simulink model "propulsionSystem"  (R2019b)
settings: Solver=VariableStepAuto  StartTime=0.0  StopTime=15.0  RelTol=1e-3
undefined symbols (not defined in the file or in its folder): sim
libraries: fl_lib x33, nesl_utility x16, SimscapeFluids_lib x1
settings Model: Creator=Edward  LastModifiedBy=Edward

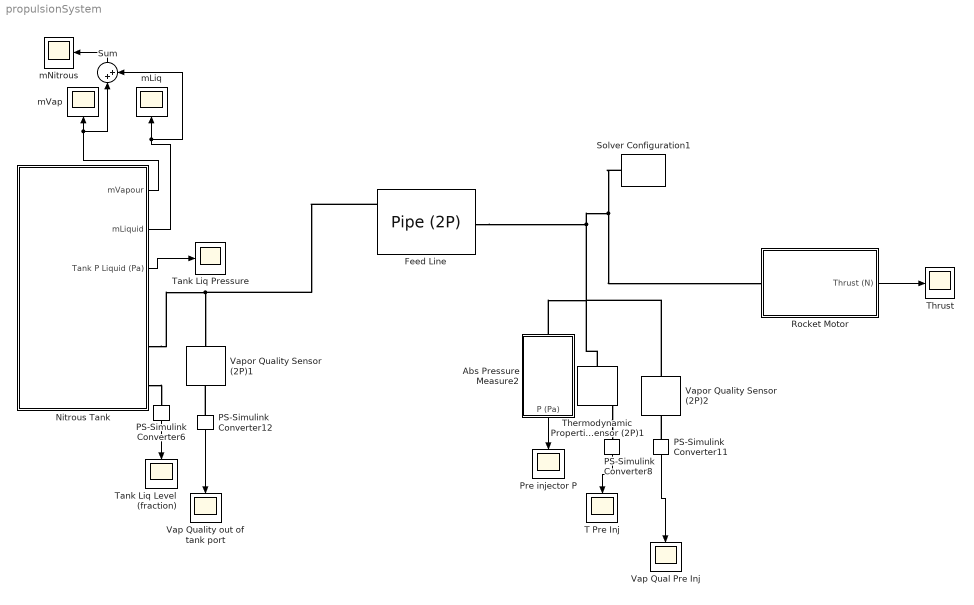
== system propulsionSystem ==
  Abs Pressure Measure2 : Subsystem
  Feed Line : fl_lib/Two-Phase Fluid/Elements/Pipe (2P)  length=10 cm  area=sim.pipe.crossSection m^2  Dh=sim.pipe.diameter m  length_add=10 cm  roughness=15e-6 m  Re_lam=2000  Re_tur=4000  shape_factor=64  Nu_lam=3.66  inertia=simscape.enum.onoff.off  energy_spec=foundation.enum.energy_spec.temperature  p_init=sim.pipe.startPressure Pa  T_init=293.15 K  x_init=0.5  alpha_init=0.5  h_init=1500 kJ/kg  u_init=1500 kJ/kg  mdot_init=0.01 kg/s  time_constant=0.1 s
      settings: SourceProductName=Simscape  SourceProductBaseCode=SS  InternalSimscapePortConfiguration="{\"Bottom\":[],\"Left\":[{\"id\":\"A\",\"label\":\"A\",\"type\":\"foundation.two_phase_fluid.two_phase_fluid\"},{\"id\":\"H\",\"label\":\"H\",\"type\":\"foundation.thermal.thermal\"}],\"Right\":[{\"id\":\"B\",\"label\":\"B\",\"type\":\"foundation.two_phase_fluid.two_phase_fluid\"}],\"Top\":[]}"
  Nitrous Tank : Subsystem
      mask Display: image('$imagefile'); % Use "Edit Image" on toolstrip to change.
  PS-Simulink Converter{6,8,11..12} (4 alike) : nesl_utility/PS-Simulink Converter  PhysicalDomain=network_engine_domain  SubClassName=ps_output  LeftPortType=input  RightPortType=output  PseudoPeriodic=off  Frequencies=[]  Unit=inherit  AffineConversion=off
  Pre injector P : Scope
  Rocket Motor : Subsystem
      mask Display: image('$imagefile'); % Use "Edit Image" on toolstrip to change.
  Solver Configuration1 : nesl_utility/Solver Configuration  PhysicalDomain=network_engine_domain  SubClassName=solver  LeftPortType=input  RightPortType=generic  Tones=[]  Harmonics=[]  SimulateNoise=off  Profile=off  UseLocalSampling=off  EnableSwitchedLinearOptims=on  FrequencyDomain=off  UseCCode=off  RelTol=0.001  AbsTol=1e-06  MinStep=1e-09  ToWorkspace=off  RevertToSquareIcSolve=off  NumHomotopyIterations=100  PhasorMode=off  PhasorModeNumHarmonics=1  DoDC=off  ResidualTolerance=1e-9  UseLocalSolver=off  LocalSolverChoice=NE_BACKWARD_EULER_ADVANCER  LocalSolverSampleTime=0.001  DoFixedCost=off  MaxNonlinIter=3  MaxModeIter=2  LinearAlgebra=auto  EquationFormulation=NE_TIME_EF  DelaysMemoryBudget=1024  AutomaticFiltering=on  FilteringTimeConstant=0.001  PartitionStorageMethod=AS_NEEDED  PartitionMemoryBudget=1024  PartitionMethod=ROBUST
  Sum : Sum  Inputs=|++
  T Pre Inj : Scope
  Tank Liq Level (fraction) : Scope
  Tank Liq Pressure : Scope
  Thermodynamic Properties Sensor (2P)1 : fl_lib/Two-Phase Fluid/Sensors/Thermodynamic Properties Sensor (2P)
      settings: SourceProductName=Simscape  SourceProductBaseCode=SS  InternalSimscapePortConfiguration="{\"Bottom\":[],\"Left\":[{\"id\":\"A\",\"label\":\"A\",\"type\":\"foundation.two_phase_fluid.two_phase_fluid\"}],\"Right\":[{\"id\":\"T\",\"label\":\"T\",\"type\":\"output\"},{\"id\":\"H\",\"label\":\"h\",\"type\":\"output\"},{\"id\":\"V\",\"label\":\"v\",\"type\":\"output\"},{\"id\":\"S\",\"label\":\"s\",\"type\":\"output\"}],\"Top\":[]}"
  Thrust : Scope
  "Vap Qual Pre Inj " : Scope
  Vap Quality out of tank port : Scope
  Vapor Quality Sensor (2P)1 : fl_lib/Two-Phase Fluid/Sensors/Vapor Quality Sensor (2P)  vapor_fraction_spec=foundation.enum.vapor_fraction_spec.quality
      settings: SourceProductName=Simscape  SourceProductBaseCode=SS  InternalSimscapePortConfiguration="{\"Bottom\":[],\"Left\":[{\"id\":\"A\",\"label\":\"A\",\"type\":\"foundation.two_phase_fluid.two_phase_fluid\"}],\"Right\":[{\"id\":\"X\",\"label\":\"X\",\"type\":\"output\"}],\"Top\":[]}"
  Vapor Quality Sensor (2P)2 : fl_lib/Two-Phase Fluid/Sensors/Vapor Quality Sensor (2P)  vapor_fraction_spec=foundation.enum.vapor_fraction_spec.quality
      settings: SourceProductName=Simscape  SourceProductBaseCode=SS  InternalSimscapePortConfiguration="{\"Bottom\":[],\"Left\":[{\"id\":\"A\",\"label\":\"A\",\"type\":\"foundation.two_phase_fluid.two_phase_fluid\"}],\"Right\":[{\"id\":\"X\",\"label\":\"X\",\"type\":\"output\"}],\"Top\":[]}"
  mLiq : Scope
  mNitrous : Scope
  mVap : Scope
  wires:
  Sum/1 -> mNitrous/1
  Nitrous Tank/1(mVapour) -> Sum/1, mVap/1
  Nitrous Tank/2(mLiquid) -> mLiq/1, Sum/2
  PS-Simulink Converter6/1 -> Tank Liq Level (fraction)/1
  Abs Pressure Measure2/1(P (Pa)) -> Pre injector P/1
  PS-Simulink Converter8/1 -> T Pre Inj/1
  PS-Simulink Converter11/1 -> "Vap Qual Pre Inj "/1
  PS-Simulink Converter12/1 -> Vap Quality out of tank port/1
  Nitrous Tank/3(Tank P Liquid (Pa)) -> Tank Liq Pressure/1
  Rocket Motor/1(Thrust (N)) -> Thrust/1
  connections:
  Thermodynamic Properties Sensor (2P)1/LConn1 -- Vapor Quality Sensor (2P)2/LConn1 -- Abs Pressure Measure2/LConn1 -- Feed Line/RConn1 -- Rocket Motor/LConn1 -- Solver Configuration1/RConn1
  Nitrous Tank/RConn3 -- PS-Simulink Converter6/LConn1
  Thermodynamic Properties Sensor (2P)1/RConn1 -- PS-Simulink Converter8/LConn1
  PS-Simulink Converter11/LConn1 -- Vapor Quality Sensor (2P)2/RConn1
  PS-Simulink Converter12/LConn1 -- Vapor Quality Sensor (2P)1/RConn1
  Nitrous Tank/RConn2 -- Feed Line/LConn1 -- Vapor Quality Sensor (2P)1/LConn1

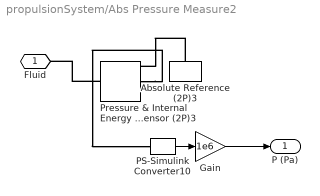
== system propulsionSystem/Abs Pressure Measure2 ==
  Absolute Reference (2P)3 : fl_lib/Two-Phase Fluid/Elements/Absolute Reference (2P)
      settings: SourceProductName=Simscape  SourceProductBaseCode=SS
  Gain : Gain  Gain=1e6
  PS-Simulink Converter10 : nesl_utility/PS-Simulink Converter  PhysicalDomain=network_engine_domain  SubClassName=ps_output  LeftPortType=input  RightPortType=output  PseudoPeriodic=off  Frequencies=[]  Unit=inherit  AffineConversion=off
  Pressure & Internal Energy Sensor (2P)3 : fl_lib/Two-Phase Fluid/Sensors/Pressure & Internal Energy Sensor (2P)
      settings: SourceProductName=Simscape  SourceProductBaseCode=SS  InternalSimscapePortConfiguration="{\"Bottom\":[],\"Left\":[{\"id\":\"A\",\"label\":\"A\",\"type\":\"foundation.two_phase_fluid.two_phase_fluid\"}],\"Right\":[{\"id\":\"B\",\"label\":\"B\",\"type\":\"foundation.two_phase_fluid.two_phase_fluid\"},{\"id\":\"P\",\"label\":\"P\",\"type\":\"output\"},{\"id\":\"U\",\"label\":\"U\",\"type\":\"output\"}],\"Top\":[]}"
  Fluid : PMIOPort  Side=Left
  P (Pa) : Outport
  wires:
  PS-Simulink Converter10/1 -> Gain/1
  Gain/1 -> P (Pa)/1
  connections:
  Absolute Reference (2P)3/LConn1 -- Pressure & Internal Energy Sensor (2P)3/RConn1
  Pressure & Internal Energy Sensor (2P)3/RConn2 -- PS-Simulink Converter10/LConn1
  Pressure & Internal Energy Sensor (2P)3/LConn1 -- Fluid/RConn1

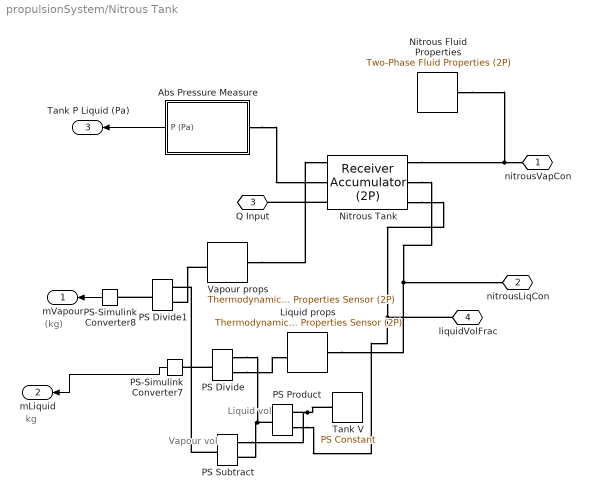
== system propulsionSystem/Nitrous Tank ==
  note: kg
  note: (kg)
  note: Vapour vol
  note: Liquid vol
  Abs Pressure Measure : Subsystem
  Liquid props : fl_lib/Two-Phase Fluid/Sensors/Thermodynamic Properties Sensor (2P)
      settings: SourceProductName=Simscape  SourceProductBaseCode=SS  InternalSimscapePortConfiguration="{\"Bottom\":[],\"Left\":[{\"id\":\"A\",\"label\":\"A\",\"type\":\"foundation.two_phase_fluid.two_phase_fluid\"}],\"Right\":[{\"id\":\"T\",\"label\":\"T\",\"type\":\"output\"},{\"id\":\"H\",\"label\":\"h\",\"type\":\"output\"},{\"id\":\"V\",\"label\":\"v\",\"type\":\"output\"},{\"id\":\"S\",\"label\":\"s\",\"type\":\"output\"}],\"Top\":[]}"
  Nitrous Fluid Properties : fl_lib/Two-Phase Fluid/Utilities/Two-Phase Fluid Properties (2P)  u_min=sim.nitrousFluidTable.u_min kJ/kg  u_max=sim.nitrousFluidTable.u_max kJ/kg  unorm_liq=sim.nitrousFluidTable.liquid.unorm  unorm_vap=sim.nitrousFluidTable.vapor.unorm  p_TLU=sim.nitrousFluidTable.p MPa  v_liq=sim.nitrousFluidTable.liquid.v m^3/kg  v_vap=sim.nitrousFluidTable.vapor.v m^3/kg  s_liq=sim.nitrousFluidTable.liquid.s kJ/kg/K  s_vap=sim.nitrousFluidTable.vapor.s kJ/kg/K  T_liq=sim.nitrousFluidTable.liquid.T K  T_vap=sim.nitrousFluidTable.vapor.T K  nu_liq=sim.nitrousFluidTable.liquid.nu mm^2/s  nu_vap=sim.nitrousFluidTable.vapor.nu mm^2/s  k_liq=sim.nitrousFluidTable.liquid.k W/(m*K)  k_vap=sim.nitrousFluidTable.vapor.k W/(m*K)  Pr_liq=sim.nitrousFluidTable.liquid.Pr  Pr_vap=sim.nitrousFluidTable.vapor.Pr  u_sat_liq=sim.nitrousFluidTable.liquid.u_sat kJ/kg  u_sat_vap=sim.nitrousFluidTable.vapor.u_sat kJ/kg  p_crit=sim.nitrousFluidTable.p_crit MPa  critical_region=foundation.enum.critical_region.clip  p_crit_fraction=0.12  p_atm=0.101325 MPa  q_rev=0.01 Pa
      settings: SourceProductName=Simscape  SourceProductBaseCode=SS  InternalSimscapePortConfiguration="{\"Bottom\":[],\"Left\":[],\"Right\":[{\"id\":\"A\",\"label\":\"\",\"type\":\"foundation.two_phase_fluid.two_phase_fluid\"}],\"Top\":[]}"
  Nitrous Tank : SimscapeFluids_lib/Two-Phase Fluid/Tanks & Accumulators/Receiver Accumulator (2P)  volume=sim.runTank.volume m^3  area_AV=2e-5 m^2  area_BV=2e-5 m^2  area_AL=2e-5 m^2  area_BL=sim.pipe.crossSection m^2  V_frac_error=simscape.enum.assert.action.none  V_frac_min=0.05  V_frac_max=0.95  V_frac_smooth=0.04  p_crit_error=simscape.enum.assert.action.error  hc_vap=20 W/(m^2 * K)  hc_liq=100 W/(m^2 * K)  surface_area=6 m^2  receiver_accumulator_energy_spec=fluids.two_phase_fluid.enum.receiver_accumulator_energy_spec.mass_fraction  p_init=64 bar  T_init=293.15 K  M_frac_init=0.7  V_frac_init=0.55  h_init=1500 kJ/kg  u_init=1500 kJ/kg  tau_vap_cond=0.1 s
      settings: SourceProductName=Simscape Fluids  SourceProductBaseCode=SH  InternalSimscapePortConfiguration="{\"Bottom\":[],\"Left\":[{\"id\":\"AV\",\"label\":\"AV\",\"type\":\"foundation.two_phase_fluid.two_phase_fluid\"},{\"id\":\"AL\",\"label\":\"AL\",\"type\":\"foundation.two_phase_fluid.two_phase_fluid\"},{\"id\":\"H\",\"label\":\"H\",\"type\":\"foundation.thermal.thermal\"}],\"Right\":[{\"id\":\"BV\",\"label\":\"BV\",\"type\":\"foundation.two_phase_fluid.two_phase_fluid\"},{\"id\":\"BL\",\"label\":\"BL\",\"type\":\"foundation.two_phase_fluid.two_phase_fluid\"},{\"id\":\"L\",\"label\":\"L\",\"type\":\"output\"}],\"Top\":[]}"
  PS Divide : fl_lib/Physical Signals/Functions/PS Divide
      settings: SourceProductName=Simscape  SourceProductBaseCode=SS
  PS Divide1 : fl_lib/Physical Signals/Functions/PS Divide
      settings: SourceProductName=Simscape  SourceProductBaseCode=SS
  PS Product : fl_lib/Physical Signals/Functions/PS Product
      settings: SourceProductName=Simscape
  PS Subtract : fl_lib/Physical Signals/Functions/PS Subtract
      settings: SourceProductName=Simscape
  PS-Simulink Converter7 : nesl_utility/PS-Simulink Converter  PhysicalDomain=network_engine_domain  SubClassName=ps_output  LeftPortType=input  RightPortType=output  PseudoPeriodic=off  Frequencies=[]  Unit=inherit  AffineConversion=off
  PS-Simulink Converter8 : nesl_utility/PS-Simulink Converter  PhysicalDomain=network_engine_domain  SubClassName=ps_output  LeftPortType=input  RightPortType=output  PseudoPeriodic=off  Frequencies=[]  Unit=inherit  AffineConversion=off
  "Tank V " : fl_lib/Physical Signals/Sources/PS Constant  constant=sim.runTank.volume m^3
  Vapour props : fl_lib/Two-Phase Fluid/Sensors/Thermodynamic Properties Sensor (2P)
      settings: SourceProductName=Simscape  SourceProductBaseCode=SS  InternalSimscapePortConfiguration="{\"Bottom\":[],\"Left\":[{\"id\":\"A\",\"label\":\"A\",\"type\":\"foundation.two_phase_fluid.two_phase_fluid\"}],\"Right\":[{\"id\":\"T\",\"label\":\"T\",\"type\":\"output\"},{\"id\":\"H\",\"label\":\"h\",\"type\":\"output\"},{\"id\":\"V\",\"label\":\"v\",\"type\":\"output\"},{\"id\":\"S\",\"label\":\"s\",\"type\":\"output\"}],\"Top\":[]}"
  nitrousVapCon : PMIOPort  Side=Right
  nitrousLiqCon : PMIOPort  Port=2  Side=Right
  Q Input : PMIOPort  Port=3  Side=Left
  liquidVolFrac : PMIOPort  Port=4  Side=Right
  mVapour : Outport
  mLiquid : Outport  Port=2
  Tank P Liquid (Pa) : Outport  Port=3
  wires:
  PS-Simulink Converter7/1 -> mLiquid/1
  PS-Simulink Converter8/1 -> mVapour/1
  Abs Pressure Measure/1(P (Pa)) -> Tank P Liquid (Pa)/1
  connections:
  Liquid props/LConn1 -- Nitrous Tank/RConn2 -- nitrousLiqCon/RConn1
  Vapour props/RConn3 -- PS Divide1/LConn2
  Nitrous Tank/RConn3 -- PS Product/LConn2 -- liquidVolFrac/RConn1
  PS Divide/RConn1 -- PS-Simulink Converter7/LConn1
  PS Product/RConn1 -- PS Divide/LConn1 -- PS Subtract/LConn2
  PS Subtract/RConn1 -- PS Divide1/LConn1
  Vapour props/LConn1 -- Nitrous Tank/LConn1
  "Tank V "/RConn1 -- PS Subtract/LConn1 -- PS Product/LConn1
  PS Divide/LConn2 -- Liquid props/RConn3
  PS Divide1/RConn1 -- PS-Simulink Converter8/LConn1
  Nitrous Tank/RConn1 -- Nitrous Fluid Properties/RConn1 -- nitrousVapCon/RConn1
  Nitrous Tank/LConn3 -- Q Input/RConn1
  Abs Pressure Measure/LConn1 -- Nitrous Tank/LConn2

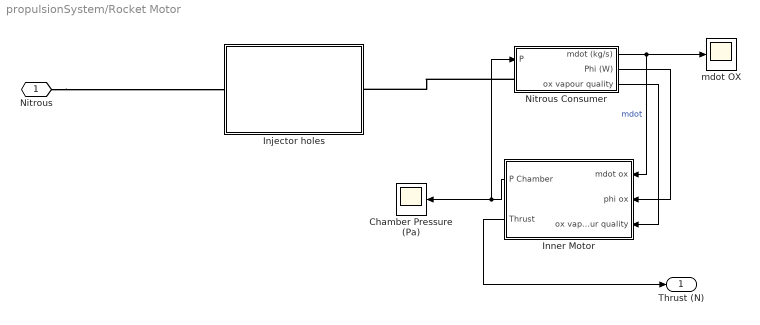
== system propulsionSystem/Rocket Motor ==
  Chamber Pressure (Pa) : Scope
  Injector holes : Subsystem
  Inner Motor : Subsystem
      mask Display: image('$imagefile'); % Use "Edit Image" on toolstrip to change.
  Nitrous Consumer : Subsystem
  mdot OX : Scope
  Nitrous : PMIOPort  Side=Left
  Thrust (N) : Outport
  wires:
  Nitrous Consumer/1(mdot (kg/s)) -> Inner Motor/1(mdot ox), mdot OX/1  "mdot"
  Inner Motor/1(P Chamber) -> Nitrous Consumer/1(P), Chamber Pressure (Pa)/1
  Nitrous Consumer/2(Phi (W)) -> Inner Motor/2(phi ox)
  Inner Motor/2(Thrust) -> Thrust (N)/1
  Nitrous Consumer/3(ox vapour quality) -> Inner Motor/3(ox vapour quality)
  connections:
  Nitrous Consumer/LConn1 -- Injector holes/RConn1
  Nitrous/RConn1 -- Injector holes/LConn1

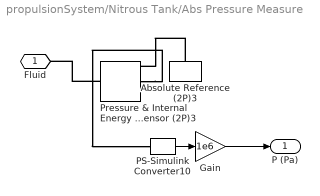
== system propulsionSystem/Nitrous Tank/Abs Pressure Measure ==
  Absolute Reference (2P)3 : fl_lib/Two-Phase Fluid/Elements/Absolute Reference (2P)
      settings: SourceProductName=Simscape  SourceProductBaseCode=SS
  Gain : Gain  Gain=1e6
  PS-Simulink Converter10 : nesl_utility/PS-Simulink Converter  PhysicalDomain=network_engine_domain  SubClassName=ps_output  LeftPortType=input  RightPortType=output  PseudoPeriodic=off  Frequencies=[]  Unit=inherit  AffineConversion=off
  Pressure & Internal Energy Sensor (2P)3 : fl_lib/Two-Phase Fluid/Sensors/Pressure & Internal Energy Sensor (2P)
      settings: SourceProductName=Simscape  SourceProductBaseCode=SS  InternalSimscapePortConfiguration="{\"Bottom\":[],\"Left\":[{\"id\":\"A\",\"label\":\"A\",\"type\":\"foundation.two_phase_fluid.two_phase_fluid\"}],\"Right\":[{\"id\":\"B\",\"label\":\"B\",\"type\":\"foundation.two_phase_fluid.two_phase_fluid\"},{\"id\":\"P\",\"label\":\"P\",\"type\":\"output\"},{\"id\":\"U\",\"label\":\"U\",\"type\":\"output\"}],\"Top\":[]}"
  Fluid : PMIOPort  Side=Left
  P (Pa) : Outport
  wires:
  PS-Simulink Converter10/1 -> Gain/1
  Gain/1 -> P (Pa)/1
  connections:
  Absolute Reference (2P)3/LConn1 -- Pressure & Internal Energy Sensor (2P)3/RConn1
  Pressure & Internal Energy Sensor (2P)3/RConn2 -- PS-Simulink Converter10/LConn1
  Pressure & Internal Energy Sensor (2P)3/LConn1 -- Fluid/RConn1

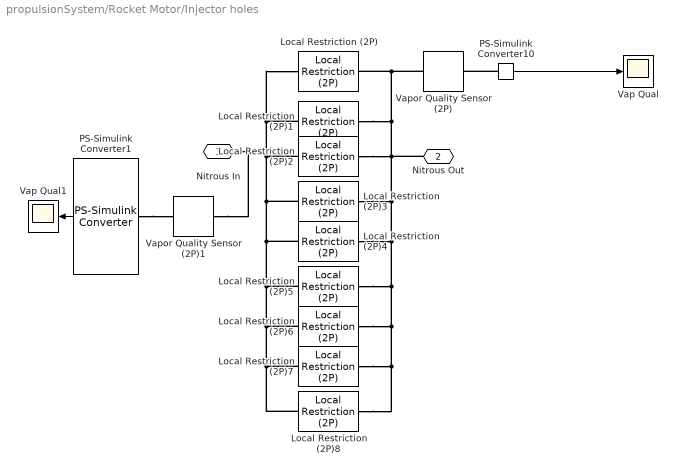
== system propulsionSystem/Rocket Motor/Injector holes ==
  Local Restriction (2P){,1..8} (9 alike) : fl_lib/Two-Phase Fluid/Elements/Local Restriction (2P)  restriction_area=sim.injector.singleHoleA m^2  area=sim.preInjectorPipe.diameter m^2  Cd=0.64  B_lam=0.999
      settings: SourceProductName=Simscape  SourceProductBaseCode=SS  InternalSimscapePortConfiguration="{\"Bottom\":[],\"Left\":[{\"id\":\"A\",\"label\":\"A\",\"type\":\"foundation.two_phase_fluid.two_phase_fluid\"}],\"Right\":[{\"id\":\"B\",\"label\":\"B\",\"type\":\"foundation.two_phase_fluid.two_phase_fluid\"}],\"Top\":[]}"
  PS-Simulink Converter1 : nesl_utility/PS-Simulink Converter  PhysicalDomain=network_engine_domain  SubClassName=ps_output  LeftPortType=input  RightPortType=output  PseudoPeriodic=off  Frequencies=[]  Unit=inherit  AffineConversion=off
  PS-Simulink Converter10 : nesl_utility/PS-Simulink Converter  PhysicalDomain=network_engine_domain  SubClassName=ps_output  LeftPortType=input  RightPortType=output  PseudoPeriodic=off  Frequencies=[]  Unit=inherit  AffineConversion=off
  Vap Qual : Scope
  Vap Qual1 : Scope
  Vapor Quality Sensor (2P) : fl_lib/Two-Phase Fluid/Sensors/Vapor Quality Sensor (2P)  vapor_fraction_spec=foundation.enum.vapor_fraction_spec.quality
      settings: SourceProductName=Simscape  SourceProductBaseCode=SS  InternalSimscapePortConfiguration="{\"Bottom\":[],\"Left\":[{\"id\":\"A\",\"label\":\"A\",\"type\":\"foundation.two_phase_fluid.two_phase_fluid\"}],\"Right\":[{\"id\":\"X\",\"label\":\"X\",\"type\":\"output\"}],\"Top\":[]}"
  Vapor Quality Sensor (2P)1 : fl_lib/Two-Phase Fluid/Sensors/Vapor Quality Sensor (2P)  vapor_fraction_spec=foundation.enum.vapor_fraction_spec.quality
      settings: SourceProductName=Simscape  SourceProductBaseCode=SS  InternalSimscapePortConfiguration="{\"Bottom\":[],\"Left\":[{\"id\":\"A\",\"label\":\"A\",\"type\":\"foundation.two_phase_fluid.two_phase_fluid\"}],\"Right\":[{\"id\":\"X\",\"label\":\"X\",\"type\":\"output\"}],\"Top\":[]}"
  Nitrous In : PMIOPort  Side=Left
  Nitrous Out : PMIOPort  Port=2  Side=Right
  wires:
  PS-Simulink Converter10/1 -> Vap Qual/1
  PS-Simulink Converter1/1 -> Vap Qual1/1
  connections:
  Nitrous Out/RConn1 -- Local Restriction (2P)8/RConn1 -- Local Restriction (2P)7/RConn1 -- Local Restriction (2P)6/RConn1 -- Local Restriction (2P)5/RConn1 -- Local Restriction (2P)4/RConn1 -- Local Restriction (2P)3/RConn1 -- Local Restriction (2P)1/RConn1 -- Vapor Quality Sensor (2P)/LConn1 -- Local Restriction (2P)/RConn1 -- Local Restriction (2P)2/RConn1
  Nitrous In/RConn1 -- Vapor Quality Sensor (2P)1/LConn1 -- Local Restriction (2P)8/LConn1 -- Local Restriction (2P)7/LConn1 -- Local Restriction (2P)6/LConn1 -- Local Restriction (2P)5/LConn1 -- Local Restriction (2P)4/LConn1 -- Local Restriction (2P)3/LConn1 -- Local Restriction (2P)2/LConn1 -- Local Restriction (2P)1/LConn1 -- Local Restriction (2P)/LConn1
  PS-Simulink Converter10/LConn1 -- Vapor Quality Sensor (2P)/RConn1
  PS-Simulink Converter1/LConn1 -- Vapor Quality Sensor (2P)1/RConn1

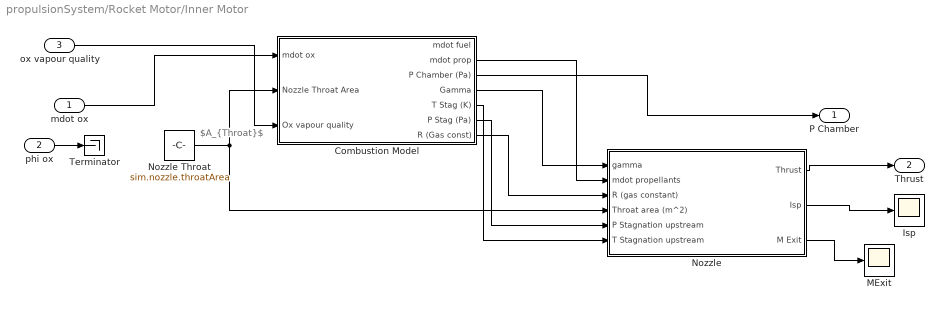
== system propulsionSystem/Rocket Motor/Inner Motor ==
  note: $A_{Throat}$
  mdot ox : Inport
  phi ox : Inport  Port=2
  ox vapour quality : Inport  Port=3
  Combustion Model : Subsystem
  Isp : Scope
  MExit : Scope
  Nozzle : Subsystem
  Nozzle Throat : Constant  Value=sim.nozzle.throatArea
  Terminator : Terminator
  P Chamber : Outport
  Thrust : Outport  Port=2
  wires:
  mdot ox/1 -> Combustion Model/1(mdot ox)
  Combustion Model/3(P Chamber (Pa)) -> P Chamber/1
  Nozzle Throat/1 -> Combustion Model/2(Nozzle Throat Area), Nozzle/4(Throat area (m^2))
  Combustion Model/4(Gamma) -> Nozzle/1(gamma)
  Combustion Model/2("mdot prop ") -> Nozzle/2(mdot propellants)
  Combustion Model/7(R (Gas const)) -> Nozzle/3(R (gas constant))
  Combustion Model/6("P Stag (Pa) ") -> Nozzle/5(P Stagnation upstream)
  Nozzle/1(Thrust) -> Thrust/1
  Nozzle/2(Isp) -> Isp/1
  Nozzle/3(M Exit) -> MExit/1
  phi ox/1 -> Terminator/1
  Combustion Model/5(T Stag (K)) -> Nozzle/6(T Stagnation upstream)
  ox vapour quality/1 -> Combustion Model/3(Ox vapour quality)

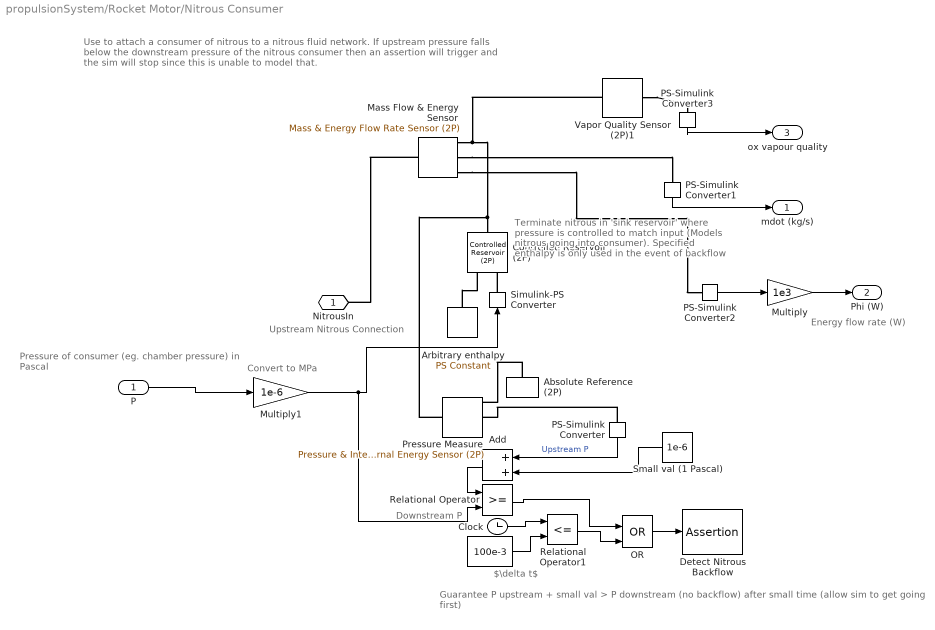
== system propulsionSystem/Rocket Motor/Nitrous Consumer ==
  note: $\delta t$
  note: Use to attach a consumer of nitrous to a nitrous fluid network.
      |
      | If upstream pressure falls below the downstream pressure of the nitrous
      | consumer then an assertion will trigger and the sim will stop since
      | this is unable to model that.
  note: Convert to MPa
  note: Terminate nitrous in 'sink reservoir'
      | where pressure is controlled to
      | match input (Models nitrous going into
      | consumer). Specified enthalpy is only used
      | in the event of backflow
  note: Guarantee P upstream + small val > P downstream (no backflow) after small time (allow sim to get going first)
  note: Downstream P
  note: Energy flow rate (W)
  note: Upstream Nitrous Connection
  note: Pressure of consumer (eg. chamber pressure)
      | in Pascal
  P : Inport
  " " : Constant  Value=100e-3
  Absolute Reference (2P) : fl_lib/Two-Phase Fluid/Elements/Absolute Reference (2P)
      settings: SourceProductName=Simscape  SourceProductBaseCode=SS
  Add : Sum
  Arbitrary enthalpy : fl_lib/Physical Signals/Sources/PS Constant  constant=362 kJ/kg
  Clock : Clock
  Controlled Reservoir (2P) : fl_lib/Two-Phase Fluid/Elements/Controlled Reservoir (2P)  energy_spec=foundation.enum.enthalpy_internal_energy_spec.enthalpy  area_A=sim.injector.postInjectorCrossSection m^2
      settings: SourceProductName=Simscape  SourceProductBaseCode=SS  InternalSimscapePortConfiguration="{\"Bottom\":[],\"Left\":[{\"id\":\"A\",\"label\":\"A\",\"type\":\"foundation.two_phase_fluid.two_phase_fluid\"}],\"Right\":[{\"id\":\"H\",\"label\":\"H\",\"type\":\"input\"},{\"id\":\"P\",\"label\":\"P\",\"type\":\"input\"}],\"Top\":[]}"
  Detect Nitrous Backflow : Assertion
  Mass Flow & Energy Sensor : fl_lib/Two-Phase Fluid/Sensors/Mass & Energy Flow Rate Sensor (2P)
      settings: SourceProductName=Simscape  SourceProductBaseCode=SS  InternalSimscapePortConfiguration="{\"Bottom\":[],\"Left\":[{\"id\":\"A\",\"label\":\"A\",\"type\":\"foundation.two_phase_fluid.two_phase_fluid\"}],\"Right\":[{\"id\":\"B\",\"label\":\"B\",\"type\":\"foundation.two_phase_fluid.two_phase_fluid\"},{\"id\":\"M\",\"label\":\"M\",\"type\":\"output\"},{\"id\":\"PHI\",\"label\":\"Phi\",\"type\":\"output\"}],\"Top\":[]}"
  Multiply : Gain  Gain=1e3
  Multiply1 : Gain  Gain=1e-6
  OR : Logic  Operator=OR  IconShape=distinctive  AllPortsSameDT=off  OutDataTypeStr=boolean
  PS-Simulink Converter{,1..3} (4 alike) : nesl_utility/PS-Simulink Converter  PhysicalDomain=network_engine_domain  SubClassName=ps_output  LeftPortType=input  RightPortType=output  PseudoPeriodic=off  Frequencies=[]  Unit=inherit  AffineConversion=off
  Pressure Measure : fl_lib/Two-Phase Fluid/Sensors/Pressure & Internal Energy Sensor (2P)
      settings: SourceProductName=Simscape  SourceProductBaseCode=SS  InternalSimscapePortConfiguration="{\"Bottom\":[],\"Left\":[{\"id\":\"A\",\"label\":\"A\",\"type\":\"foundation.two_phase_fluid.two_phase_fluid\"}],\"Right\":[{\"id\":\"B\",\"label\":\"B\",\"type\":\"foundation.two_phase_fluid.two_phase_fluid\"},{\"id\":\"P\",\"label\":\"P\",\"type\":\"output\"},{\"id\":\"U\",\"label\":\"U\",\"type\":\"output\"}],\"Top\":[]}"
  Relational Operator : RelationalOperator  OutDataTypeStr=boolean  RndMeth=Simplest
  Relational Operator1 : RelationalOperator  Operator=<=  OutDataTypeStr=boolean  RndMeth=Simplest
  Simulink-PS Converter : nesl_utility/Simulink-PS Converter  PhysicalDomain=network_engine_domain  SubClassName=ps_input  LeftPortType=input  RightPortType=output  PseudoPeriodic=off  Frequencies=[]  NoiseDistribution=none  NoiseParameters=[]  Unit=1  AffineConversion=off  FilteringAndDerivatives=provide  SimscapeFilterOrder=1  InputFilterTimeConstant=0.001  UdotUserProvided=0
  Small val (1 Pascal) : Constant  Value=1e-6
  Vapor Quality Sensor (2P)1 : fl_lib/Two-Phase Fluid/Sensors/Vapor Quality Sensor (2P)  vapor_fraction_spec=foundation.enum.vapor_fraction_spec.quality
      settings: SourceProductName=Simscape  SourceProductBaseCode=SS  InternalSimscapePortConfiguration="{\"Bottom\":[],\"Left\":[{\"id\":\"A\",\"label\":\"A\",\"type\":\"foundation.two_phase_fluid.two_phase_fluid\"}],\"Right\":[{\"id\":\"X\",\"label\":\"X\",\"type\":\"output\"}],\"Top\":[]}"
  NitrousIn : PMIOPort  Side=Left
  mdot (kg/s) : Outport
  Phi (W) : Outport  Port=2
  ox vapour quality : Outport  Port=3
  wires:
  Relational Operator/1 -> OR/1
  PS-Simulink Converter1/1 -> mdot (kg/s)/1
  P/1 -> Multiply1/1
  PS-Simulink Converter2/1 -> Multiply/1
  Multiply/1 -> Phi (W)/1
  Multiply1/1 -> Relational Operator/2, Simulink-PS Converter/1
  PS-Simulink Converter3/1 -> ox vapour quality/1
  PS-Simulink Converter/1 -> Add/1  "Upstream P"
  Add/1 -> Relational Operator/1
  Small val (1 Pascal)/1 -> Add/2
  Clock/1 -> Relational Operator1/1
  " "/1 -> Relational Operator1/2
  Relational Operator1/1 -> OR/2
  OR/1 -> Detect Nitrous Backflow/1
  connections:
  Simulink-PS Converter/RConn1 -- Controlled Reservoir (2P)/RConn2
  Arbitrary enthalpy/RConn1 -- Controlled Reservoir (2P)/RConn1
  Mass Flow & Energy Sensor/RConn1 -- Vapor Quality Sensor (2P)1/LConn1 -- Pressure Measure/LConn1 -- Controlled Reservoir (2P)/LConn1
  Absolute Reference (2P)/LConn1 -- Pressure Measure/RConn1
  PS-Simulink Converter/LConn1 -- Pressure Measure/RConn2
  Mass Flow & Energy Sensor/RConn2 -- PS-Simulink Converter1/LConn1
  Mass Flow & Energy Sensor/RConn3 -- PS-Simulink Converter2/LConn1
  Mass Flow & Energy Sensor/LConn1 -- NitrousIn/RConn1
  Vapor Quality Sensor (2P)1/RConn1 -- PS-Simulink Converter3/LConn1

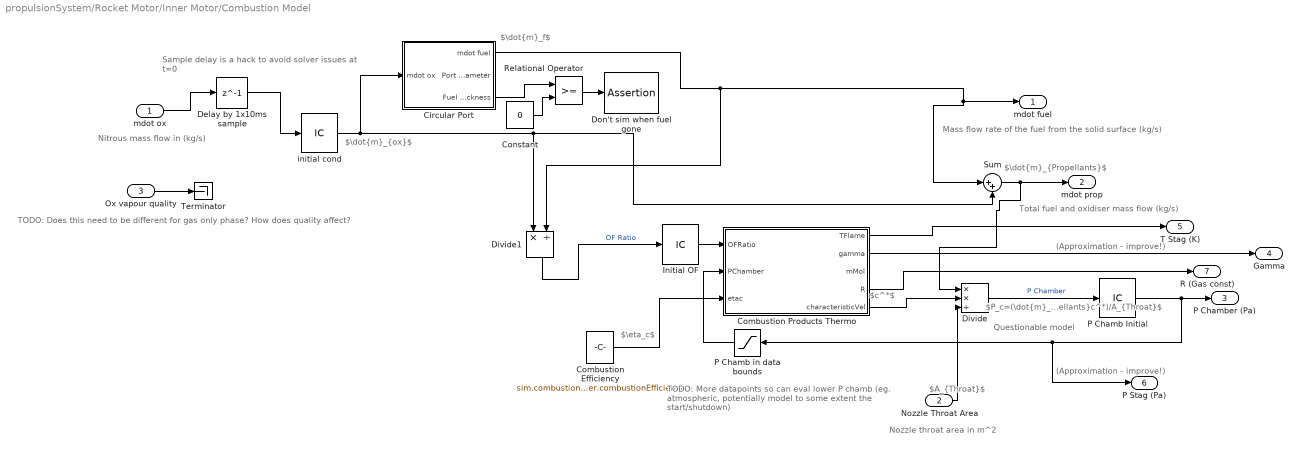
== system propulsionSystem/Rocket Motor/Inner Motor/Combustion Model ==
  note: $\eta_c$
  note: $\dot{m}_f$
  note: $\dot{m}_{ox}$
  note: $\dot{m}_{Propellants}$
  note: $A_{Throat}$
  note: $c^*$
  note: Questionable model
  note: $P_c=(\dot{m}_{propellants}c^*)/A_{Throat}$
  note: TODO: Does this need to be different for gas only phase? How does quality affect?
  note: Sample delay is a hack to avoid solver issues
      | at t=0
  note: TODO: More datapoints
      | so can eval lower P chamb (eg. atmospheric, potentially
      | model to some extent the start/shutdown)
  note: (Approximation - improve!)
  note: Total fuel and oxidiser mass flow (kg/s)
  note: Mass flow rate of the fuel from the solid surface (kg/s)
  note: Nitrous mass flow in (kg/s)
  note: Nozzle throat area in m^2
  note: (Approximation - improve!)
  mdot ox : Inport
  Nozzle Throat Area : Inport  Port=2
  Ox vapour quality : Inport  Port=3
  Circular Port : Subsystem
  Combustion Efficiency : Constant  Value=sim.combustionChamber.combustionEfficiency
  Combustion Products Thermo : MATLAB Function  TreatAsAtomicUnit=on
  Constant : Constant  Value=0
  Delay by 1x10ms sample : Delay  DelayLength=1  InitialCondition=sim.combustionChamber.mdotOxInitial  SampleTime=10e-3
  Divide : Product  Inputs=**/
  Divide1 : Product  Inputs=*/
  Don't sim when fuel gone : Assertion
  "Initial OF " : InitialCondition  Value=sim.combustionChamber.OFRatioInitial
  P Chamb Initial : InitialCondition  Value=sim.combustionChamber.PChamberInit
  P Chamb in data bounds : Saturate  UpperLimit=45e5  LowerLimit=15.1e5
  Relational Operator : RelationalOperator  OutDataTypeStr=boolean  RndMeth=Simplest
  Sum : Sum  Inputs=|++
  Terminator : Terminator
  initial cond : InitialCondition  Value=sim.combustionChamber.mdotOxInitial
  mdot fuel : Outport
  "mdot prop " : Outport  Port=2
  P Chamber (Pa) : Outport  Port=3
  Gamma : Outport  Port=4
  T Stag (K) : Outport  Port=5
  "P Stag (Pa) " : Outport  Port=6
  R (Gas const) : Outport  Port=7
  wires:
  Sum/1 -> Divide/1, "mdot prop "/1
  Combustion Products Thermo/5(characteristicVel) -> Divide/2
  Nozzle Throat Area/1 -> Divide/3
  Divide/1 -> P Chamb Initial/1  "P Chamber"
  Combustion Efficiency/1 -> Combustion Products Thermo/3(etac)
  Combustion Products Thermo/1(TFlame) -> T Stag (K)/1
  Combustion Products Thermo/2(gamma) -> Gamma/1
  Circular Port/3(Fuel web thickness) -> Relational Operator/1
  Constant/1 -> Relational Operator/2
  Relational Operator/1 -> Don't sim when fuel gone/1
  P Chamb in data bounds/1 -> Combustion Products Thermo/2(PChamber)
  Circular Port/1(mdot fuel) -> Divide1/2, Sum/1, mdot fuel/1
  "Initial OF "/1 -> Combustion Products Thermo/1(OFRatio)
  initial cond/1 -> Circular Port/1(mdot ox), Sum/2, Divide1/1
  Divide1/1 -> "Initial OF "/1  "OF Ratio"
  mdot ox/1 -> Delay by 1x10ms sample/1
  Delay by 1x10ms sample/1 -> initial cond/1
  Combustion Products Thermo/4(R) -> R (Gas const)/1
  P Chamb Initial/1 -> P Chamb in data bounds/1, "P Stag (Pa) "/1, P Chamber (Pa)/1
  Ox vapour quality/1 -> Terminator/1

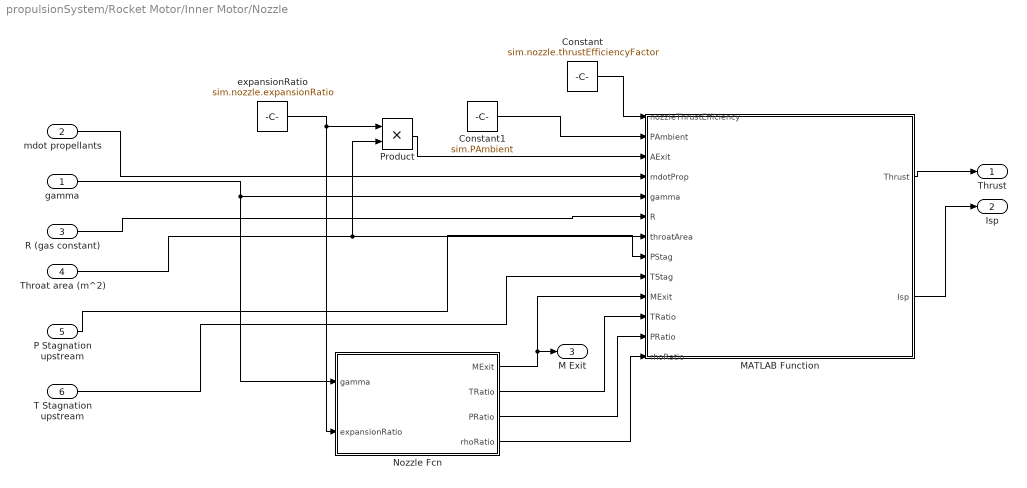
== system propulsionSystem/Rocket Motor/Inner Motor/Nozzle ==
  gamma : Inport
  mdot propellants : Inport  Port=2
  R (gas constant) : Inport  Port=3
  Throat area (m^2) : Inport  Port=4
  P Stagnation upstream : Inport  Port=5
  T Stagnation upstream : Inport  Port=6
  Constant : Constant  Value=sim.nozzle.thrustEfficiencyFactor
  Constant1 : Constant  Value=sim.PAmbient
  MATLAB Function : MATLAB Function  TreatAsAtomicUnit=on
  Nozzle Fcn : MATLAB Function  TreatAsAtomicUnit=on
  Product : Product
  "expansionRatio " : Constant  Value=sim.nozzle.expansionRatio
  Thrust : Outport
  Isp : Outport  Port=2
  M Exit : Outport  Port=3
  wires:
  gamma/1 -> Nozzle Fcn/1(gamma), MATLAB Function/5(gamma)
  "expansionRatio "/1 -> Product/1, Nozzle Fcn/2(expansionRatio)
  mdot propellants/1 -> MATLAB Function/4(mdotProp)
  R (gas constant)/1 -> MATLAB Function/6(R)
  Throat area (m^2)/1 -> Product/2, MATLAB Function/7(throatArea)
  P Stagnation upstream/1 -> MATLAB Function/8(PStag)
  Nozzle Fcn/1(MExit) -> M Exit/1, MATLAB Function/10(MExit)
  Nozzle Fcn/2(TRatio) -> MATLAB Function/11(TRatio)
  Nozzle Fcn/3(PRatio) -> MATLAB Function/12(PRatio)
  Nozzle Fcn/4(rhoRatio) -> MATLAB Function/13(rhoRatio)
  MATLAB Function/1(Thrust) -> Thrust/1
  MATLAB Function/2(Isp) -> Isp/1
  T Stagnation upstream/1 -> MATLAB Function/9(TStag)
  Constant/1 -> MATLAB Function/1(nozzleThrustEfficiency)
  Product/1 -> MATLAB Function/3(AExit)
  Constant1/1 -> MATLAB Function/2(PAmbient)

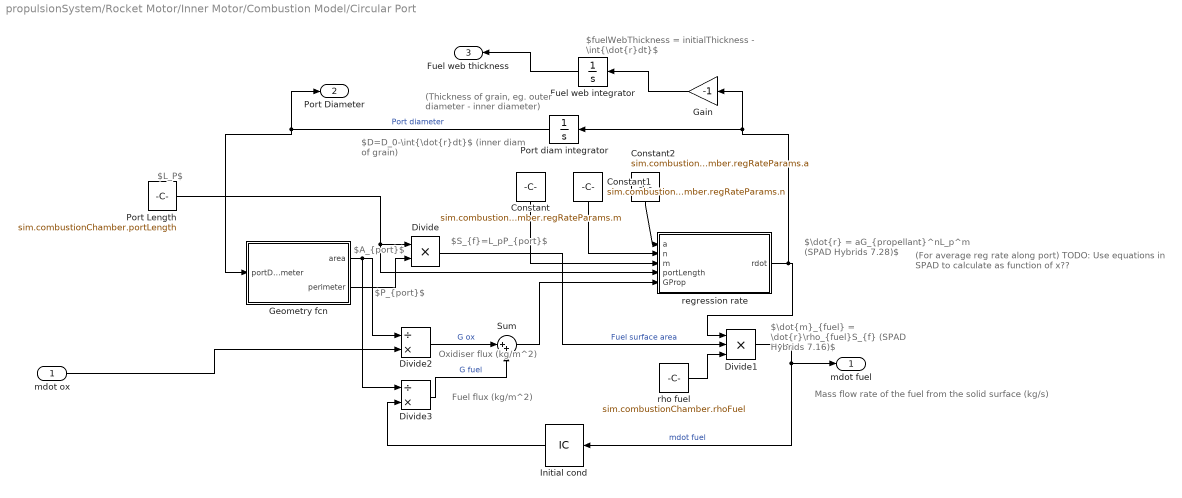
== system propulsionSystem/Rocket Motor/Inner Motor/Combustion Model/Circular Port ==
  note: $S_{f}=L_pP_{port}$
  note: $A_{port}$
  note: $P_{port}$
  note: $\dot{m}_{fuel} = \dot{r}\rho_{fuel}S_{f} (SPAD Hybrids 7.16)$
  note: Oxidiser flux (kg/m^2)
  note: (Thickness of grain, eg. outer
      | diameter - inner diameter)
  note: $fuelWebThickness = initialThickness - \int{\dot{r}dt}$
  note: $D=D_0-\int{\dot{r}dt}$ (inner diam of grain)
  note: $L_P$
  note: (For average reg rate along port)
      | TODO: Use equations in SPAD to calculate as function of
      | x??
  note: $\dot{r} = aG_{propellant}^nL_p^m (SPAD Hybrids 7.28)$
  note: Mass flow rate of the fuel from the solid surface (kg/s)
  note: Fuel flux (kg/m^2)
  mdot ox : Inport
  Constant : Constant  Value=sim.combustionChamber.regRateParams.m
  Constant1 : Constant  Value=sim.combustionChamber.regRateParams.n
  Constant2 : Constant  Value=sim.combustionChamber.regRateParams.a
  Divide : Product  Inputs=**
  Divide1 : Product  Inputs=***
  Divide2 : Product  Inputs=/*
  Divide3 : Product  Inputs=/*
  "Fuel web integrator " : Integrator  InitialCondition=sim.combustionChamber.initialFuelWebThickness
  Gain : Gain  Gain=-1
  "Geometry fcn " : MATLAB Function  TreatAsAtomicUnit=on
  Initial cond : InitialCondition  Value=sim.combustionChamber.mdotOxInitial / sim.combustionChamber.OFRatioInitial
  Port Length : Constant  Value=sim.combustionChamber.portLength
  Port diam integrator : Integrator  InitialCondition=sim.combustionChamber.initialPortDiameter
  Sum : Sum  Inputs=|++
  regression rate : MATLAB Function  TreatAsAtomicUnit=on
  rho fuel : Constant  Value=sim.combustionChamber.rhoFuel
  mdot fuel : Outport
  Port Diameter : Outport  Port=2
  Fuel web thickness : Outport  Port=3
  wires:
  Port Length/1 -> regression rate/4(portLength), Divide/1
  "Geometry fcn "/1(area) -> Divide3/1, Divide2/1
  Divide/1 -> Divide1/2  "Fuel surface area"
  rho fuel/1 -> Divide1/3
  Divide1/1 -> mdot fuel/1, Initial cond/1  "mdot fuel"
  Divide3/1 -> Sum/2  "G fuel"
  Divide2/1 -> Sum/1  "G ox"
  mdot ox/1 -> Divide2/2
  Sum/1 -> regression rate/5(GProp)
  Port diam integrator/1 -> "Geometry fcn "/1(portDiameter), Port Diameter/1  "Port diameter"
  regression rate/1(rdot) -> Gain/1, Port diam integrator/1, Divide1/1
  Gain/1 -> "Fuel web integrator "/1
  "Fuel web integrator "/1 -> Fuel web thickness/1
  Constant/1 -> regression rate/3(m)
  Constant1/1 -> regression rate/2(n)
  Constant2/1 -> regression rate/1(a)
  Initial cond/1 -> Divide3/2
  "Geometry fcn "/2(perimeter) -> Divide/2

== matlab function propulsionSystem/Rocket Motor/Inner Motor/Combustion Model/Circular Port/Geometry fcn  ==
  data: portDiameter input; area output; perimeter output
function [area, perimeter] = fcn(portDiameter)
area = pi.*(portDiameter./2).^2;
perimeter = pi.*portDiameter;

== matlab function propulsionSystem/Rocket Motor/Inner Motor/Combustion Model/Combustion Products Thermo ==
  data: OFRatio input; TFlame output; PChamber input; etac input; gamma output; mMol output; R output; characteristicVel output; propepProps parameter
function [TFlame, gamma, mMol, R, characteristicVel] = combustionProductsProperties(OFRatio, PChamber, etac, propepProps)
%Keep within data. TODO: Expand dataset
if(OFRatio > 10)
   OFRatio = 10; 
end
if(OFRatio < 2.003)
   OFRatio = 2.003; 
end
[TFlame, gamma, mMol, R, characteristicVel] = HybridMotor.thermochem(propepProps, OFRatio, PChamber, etac);

== matlab function propulsionSystem/Rocket Motor/Inner Motor/Nozzle/Nozzle Fcn ==
  data: gamma input; MExit output; expansionRatio input; TRatio output; PRatio output; rhoRatio output
function [MExit, TRatio, PRatio, rhoRatio] = nozzle(gamma, expansionRatio)
coder.extrinsic('flowisentropic'); %flowisentropic doesn't support codegen
%Initialize variables so types are determined
MExit = 0;
TRatio = 0;
PRatio = 0;
rhoRatio = 0;
[MExit, TRatio, PRatio, rhoRatio, ~] = flowisentropic(gamma, expansionRatio, 'sup');

== matlab function propulsionSystem/Rocket Motor/Inner Motor/Combustion Model/Circular Port/regression rate ==
  data: a input; n input; m input; portLength input; rdot output; GProp input
function rdot = regressionRate(a, n, m, portLength, GProp)
rdot = a.*(GProp.^n).*portLength.^m;

== matlab function propulsionSystem/Rocket Motor/Inner Motor/Nozzle/MATLAB Function ==
  data: nozzleThrustEfficiency input; PAmbient input; AExit input; Thrust output; Isp output; mdotProp input; gamma input; R input; throatArea input; PStag input; TStag input; MExit input; TRatio input; PRatio input; rhoRatio input
function [Thrust, Isp] = thrustFunction(nozzleThrustEfficiency, PAmbient, AExit, mdotProp, gamma, R, throatArea, PStag, TStag, MExit, TRatio, PRatio, rhoRatio)
TExit = TStag .* TRatio;
PExit = PStag .* PRatio;
vExit = MExit.*sqrt(gamma.*R.*TExit);
Thrust = nozzleThrustEfficiency.*(mdotProp.*vExit + (PExit-PAmbient).*AExit); %thrust
Isp = Thrust ./ (mdotProp .* 9.81);
